simulink model "compressor"  (R2012b)
settings: Solver=ode45  StartTime=0.0  StopTime=10.0  RelTol=1e-3
values from neighbouring files (symbols this model uses):
  c_p = cp_air    [Init_Project2.m]
  comp =     [turboMap.mat]
  comp_para2 = lsqcurvefit(fn2,[1 1 1 0.8 0.07 1.5], xdata, ydata)    [Init_Project2.m]
  cp_air = gamma_air*cv_air    (= 1213.33333333)    [Init_Project1.m]
  dC2 = 56e-03    (= 0.056)    [Init_Project2.m]
  gamma_air = 1.3    [Init_Project1.m]
  m_dot_c_corr_max = comp_para1(2)    [Init_Project2.m]
  p_amb = 101.3e3    (= 101300)    [Init_Project1.m]
  p_ref = comp.pCref    [Init_Project2.m]
  Psi_max = comp_para1(1)    [Init_Project2.m]
  T_amb = 293    [Init_Project1.m]
  T_ref = comp.TCref    [Init_Project2.m]
settings Model: Creator=rasme879  LastModifiedBy=adalu838
settings DataIOCC: SignalLoggingSaveFormat=ModelDataLogs
settings OptimizationCC: ExpressionDepthLimit=128
settings DebuggingCC: MultiTaskDSMMsg=warning  MultiTaskCondExecSysMsg=none  StrictBusMsg=None
settings RTWCC: IncludeERTFirstTime=on
settings CodeAppCC: CustomSymbolStrType=$N$R$M_T  InternalIdentifier=Shortened

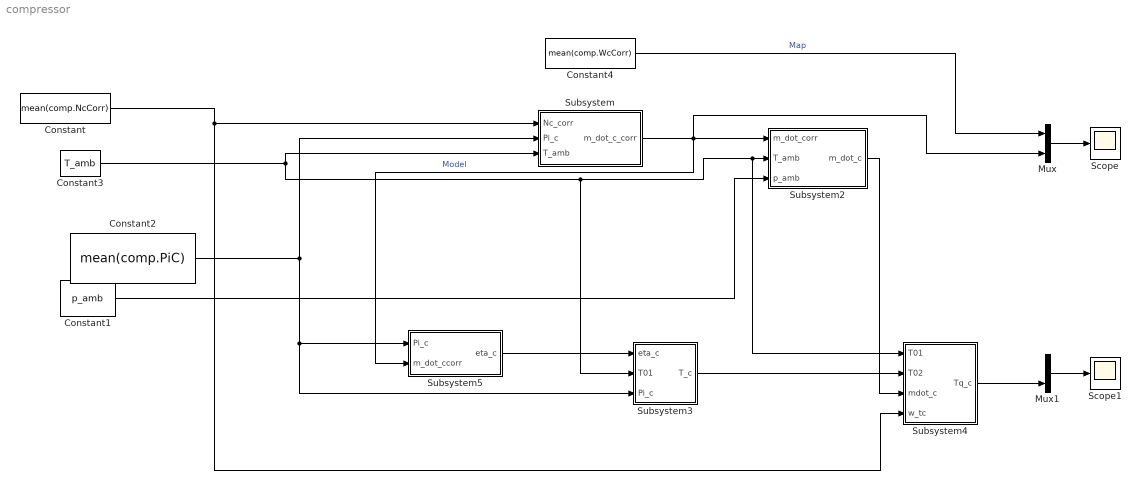
== system compressor ==
  Constant : Constant  Value=mean(comp.NcCorr)
  Constant1 : Constant  Value=p_amb
  Constant2 : Constant  Value=mean(comp.PiC)
  Constant3 : Constant  Value=T_amb
  Constant4 : Constant  Value=mean(comp.WcCorr)
  Mux : Mux  Inputs=2
  Mux1 : Mux  Inputs=2
  Scope : Scope
      settings: ShowLegends=on
  Scope1 : Scope
  Subsystem : Subsystem
  Subsystem2 : Subsystem
  Subsystem3 : Subsystem
  Subsystem4 : Subsystem
  Subsystem5 : Subsystem
  wires:
  Constant1/1 -> Subsystem2/3(p_amb)
  Constant2/1 -> Subsystem3/3(Pi_c), Subsystem5/1(Pi_c), Subsystem/2(Pi_c)
  Constant3/1 -> Subsystem3/2(T01), Subsystem4/1(T01), Subsystem2/2(T_amb), Subsystem/3(T_amb)
  Constant/1 -> Subsystem/1(Nc_corr), Subsystem4/4(w_tc)
  Subsystem/1(m_dot_c_corr) -> Mux/2, Subsystem5/2(m_dot_ccorr), Subsystem2/1(m_dot_corr)  "Model"
  Subsystem2/1(m_dot_c) -> Subsystem4/3(mdot_c)
  Subsystem4/1(Tq_c) -> Mux1/2
  Subsystem5/1(eta_c) -> Subsystem3/1(eta_c)
  Subsystem3/1(T_c) -> Subsystem4/2(T02)
  Mux/1 -> Scope/1
  Constant4/1 -> Mux/1  "Map"
  Mux1/1 -> Scope1/1

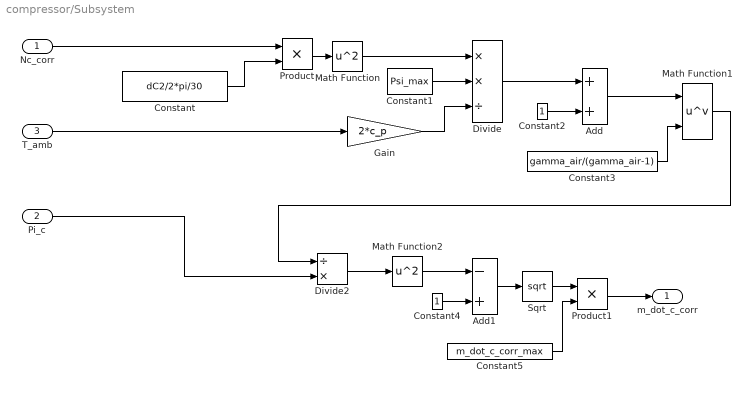
== system compressor/Subsystem ==
  Nc_corr : Inport
  Pi_c : Inport  Port=2
  T_amb : Inport  Port=3
  Add : Sum
  Add1 : Sum  Inputs=-+
  Constant : Constant  Value=dC2/2*pi/30
  Constant1 : Constant  Value=Psi_max
  Constant2 : Constant
  Constant3 : Constant  Value=gamma_air/(gamma_air-1)
  Constant4 : Constant
  Constant5 : Constant  Value=m_dot_c_corr_max
  Divide : Product  Inputs=**/
  Divide2 : Product  Inputs=/*
  Gain : Gain  Gain=2*c_p
  Math Function : Math  Operator=square  SaturateOnIntegerOverflow=on
  Math Function1 : Math  Operator=pow  SaturateOnIntegerOverflow=on
  Math Function2 : Math  Operator=square  SaturateOnIntegerOverflow=on
  Product : Product
  Product1 : Product
  Sqrt : Sqrt  SaturateOnIntegerOverflow=on
  m_dot_c_corr : Outport
  wires:
  Constant/1 -> Product/2
  Divide/1 -> Add/1
  Product1/1 -> m_dot_c_corr/1
  Product/1 -> Math Function/1
  Math Function/1 -> Divide/1
  Constant4/1 -> Add1/2
  Gain/1 -> Divide/3
  Pi_c/1 -> Divide2/2
  Math Function1/1 -> Divide2/1
  Constant1/1 -> Divide/2
  Add/1 -> Math Function1/1
  Constant5/1 -> Product1/2
  Divide2/1 -> Math Function2/1
  Add1/1 -> Sqrt/1
  Constant3/1 -> Math Function1/2
  Math Function2/1 -> Add1/1
  Nc_corr/1 -> Product/1
  Constant2/1 -> Add/2
  Sqrt/1 -> Product1/1
  T_amb/1 -> Gain/1

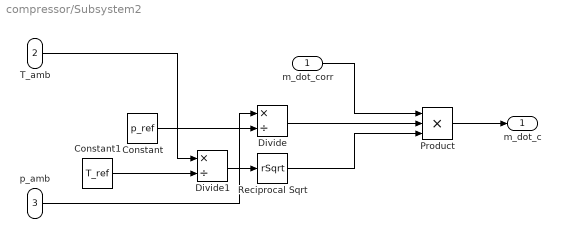
== system compressor/Subsystem2 ==
  m_dot_corr : Inport
  T_amb : Inport  Port=2
  p_amb : Inport  Port=3
  Constant : Constant  Value=p_ref
  Constant1 : Constant  Value=T_ref
  Divide : Product  Inputs=*/
  Divide1 : Product  Inputs=*/
  Product : Product  Inputs=3
  Reciprocal Sqrt : Sqrt  Operator=rSqrt  SaturateOnIntegerOverflow=on
  m_dot_c : Outport
  wires:
  T_amb/1 -> Divide1/1
  p_amb/1 -> Divide/1
  Reciprocal Sqrt/1 -> Product/3
  m_dot_corr/1 -> Product/1
  Constant/1 -> Divide/2
  Divide/1 -> Product/2
  Product/1 -> m_dot_c/1
  Divide1/1 -> Reciprocal Sqrt/1
  Constant1/1 -> Divide1/2

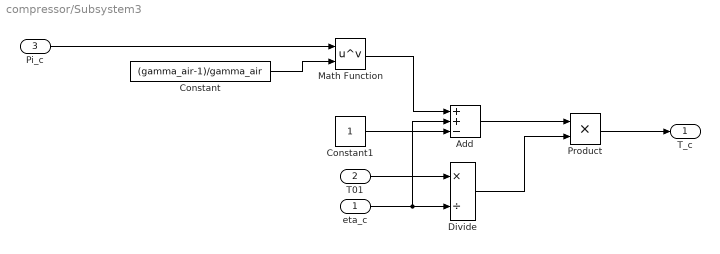
== system compressor/Subsystem3 ==
  eta_c : Inport
  T01 : Inport  Port=2
  Pi_c : Inport  Port=3
  Add : Sum  Inputs=++-
  Constant : Constant  Value=(gamma_air-1)/gamma_air
  Constant1 : Constant
  Divide : Product  Inputs=*/
  Math Function : Math  Operator=pow  SaturateOnIntegerOverflow=on
  Product : Product  RndMeth=Zero
  T_c : Outport
  wires:
  T01/1 -> Divide/1
  eta_c/1 -> Add/2, Divide/2
  Divide/1 -> Product/2
  Pi_c/1 -> Math Function/1
  Constant/1 -> Math Function/2
  Product/1 -> T_c/1
  Add/1 -> Product/1
  Constant1/1 -> Add/3
  Math Function/1 -> Add/1

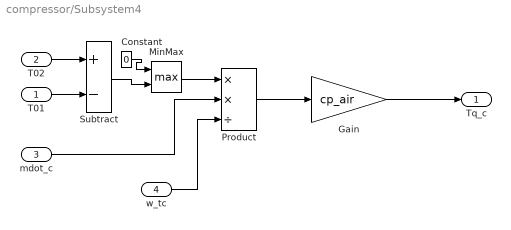
== system compressor/Subsystem4 ==
  T01 : Inport
  T02 : Inport  Port=2
  mdot_c : Inport  Port=3
  w_tc : Inport  Port=4
  Constant : Constant  Value=0
  Gain : Gain  Gain=cp_air
  MinMax : MinMax  Function=max  Inputs=2
  Product : Product  Inputs=**/  RndMeth=Zero
  Subtract : Sum  Inputs=+-
  Tq_c : Outport
  wires:
  Product/1 -> Gain/1
  Gain/1 -> Tq_c/1
  T02/1 -> Subtract/1
  T01/1 -> Subtract/2
  mdot_c/1 -> Product/2
  w_tc/1 -> Product/3
  MinMax/1 -> Product/1
  Subtract/1 -> MinMax/2
  Constant/1 -> MinMax/1

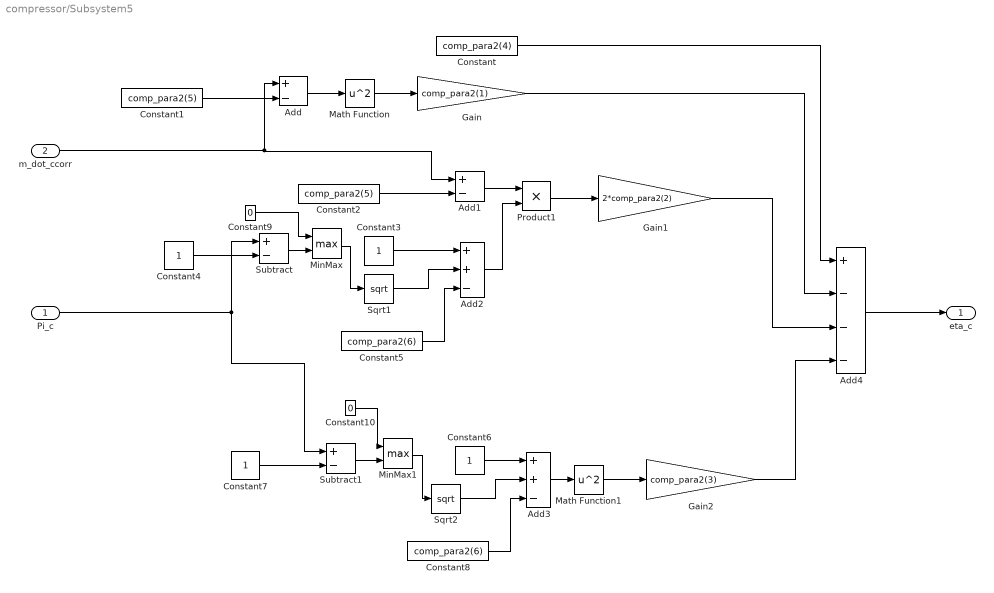
== system compressor/Subsystem5 ==
  Pi_c : Inport
  m_dot_ccorr : Inport  Port=2
  Add : Sum  Inputs=+-
  Add1 : Sum  Inputs=+-
  Add2 : Sum  Inputs=++-
  Add3 : Sum  Inputs=++-
  Add4 : Sum  Inputs=+---
  Constant : Constant  Value=comp_para2(4)
  Constant1 : Constant  Value=comp_para2(5)
  Constant10 : Constant  Value=0
  Constant2 : Constant  Value=comp_para2(5)
  Constant{3..4,6..7} (4 alike) : Constant
  Constant5 : Constant  Value=comp_para2(6)
  Constant8 : Constant  Value=comp_para2(6)
  Constant9 : Constant  Value=0
  Gain : Gain  Gain=comp_para2(1)
  Gain1 : Gain  Gain=2*comp_para2(2)
  Gain2 : Gain  Gain=comp_para2(3)
  Math Function : Math  Operator=square  SaturateOnIntegerOverflow=on
  Math Function1 : Math  Operator=square  SaturateOnIntegerOverflow=on
  MinMax : MinMax  Function=max  Inputs=2
  MinMax1 : MinMax  Function=max  Inputs=2
  Product1 : Product  RndMeth=Zero
  Sqrt1 : Sqrt  SaturateOnIntegerOverflow=on
  Sqrt2 : Sqrt  SaturateOnIntegerOverflow=on
  Subtract : Sum  Inputs=+-
  Subtract1 : Sum  Inputs=+-
  eta_c : Outport
  wires:
  Constant1/1 -> Add/2
  m_dot_ccorr/1 -> Add/1, Add1/1
  Add/1 -> Math Function/1
  Math Function/1 -> Gain/1
  Constant2/1 -> Add1/2
  Add1/1 -> Product1/1
  Product1/1 -> Gain1/1
  Add2/1 -> Product1/2
  Sqrt1/1 -> Add2/2
  Constant3/1 -> Add2/1
  Constant4/1 -> Subtract/2
  Pi_c/1 -> Subtract/1, Subtract1/1
  Constant5/1 -> Add2/3
  Sqrt2/1 -> Add3/2
  Constant6/1 -> Add3/1
  Constant7/1 -> Subtract1/2
  Constant8/1 -> Add3/3
  Add3/1 -> Math Function1/1
  Math Function1/1 -> Gain2/1
  Add4/1 -> eta_c/1
  Gain2/1 -> Add4/4
  Gain1/1 -> Add4/3
  Gain/1 -> Add4/2
  Constant/1 -> Add4/1
  Constant9/1 -> MinMax/1
  Constant10/1 -> MinMax1/1
  Subtract1/1 -> MinMax1/2
  MinMax1/1 -> Sqrt2/1
  Subtract/1 -> MinMax/2
  MinMax/1 -> Sqrt1/1
